simulink model "pll_wbsd_2"  (Simulink 7.4)
settings: Solver=ode45  StartTime=0.0  StopTime=1e-4  FixedStep=.01/(fr*N/M)  MaxStep=1/(50*fr*(N+f))  RelTol=1e-7  AbsTol=1e-4
PreLoadFcn:
  | fr=48e6,fi=2449e6,sen=200e6,N=51,f=0.125
undefined symbols (not defined in the file or in its folder): One, sen, sided
libraries: dspsigops x5, simulink_extras x2, dspswit3 x1, simulink x1, dspsnks4 x1, dsparch4 x1, commsynccomp2 x1
settings Model: Creator=Owner  LastModifiedBy=dbenson  SimulationMode=accelerator  BufferReuse=off
settings DataIOCC: LimitDataPoints=off  SaveOutput=off  SaveTime=off  SignalLoggingName=sigsOut
settings OptimizationCC: BlockReduction=off  BooleanDataType=off  InlineInvariantSignals=on  OptimizeBlockIOStorage=off  BufferReuse=off  ExpressionFolding=off  LocalBlockOutputs=off  InitFltsAndDblsToZero=on
settings DebuggingCC: SaveWithParameterizedLinksMsg=none  SignalResolutionControl=TryResolveAllWithWarning  SolverPrmCheckMsg=none  MultiTaskDSMMsg=warning  MultiTaskCondExecSysMsg=none  StrictBusMsg=None
settings HardwareCC: TargetUnknown=on
settings RTWCC: IncludeERTFirstTime=on
settings GRTTargetCC: TargetFcnLib=ansi_tfl_tmw.mat

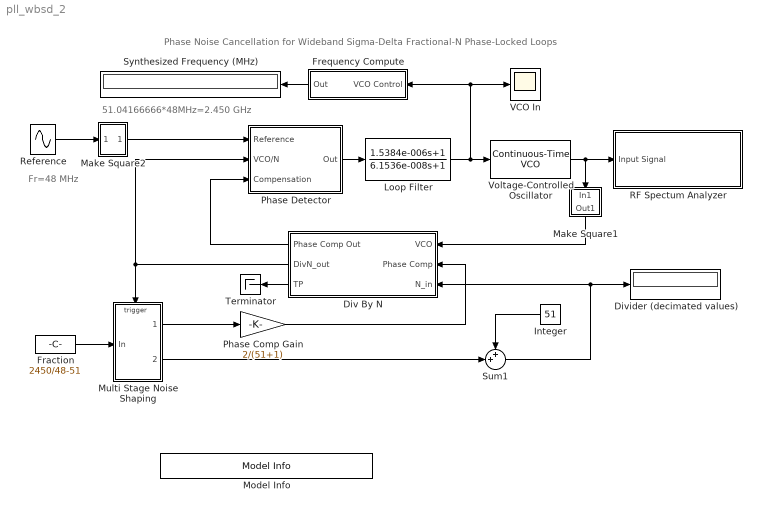
== system pll_wbsd_2 ==
  note: Phase Noise Cancellation for Wideband Sigma-Delta Fractional-N Phase-Locked Loops
  note: Fr=48 MHz
  note: 51.04166666*48MHz=2.450 GHz
  Div By N : Subsystem
  Divider (decimated values) : Display
      settings: Decimation=100
  Fraction : Constant  Value=2450/48-51  OutDataType=sfix(16)  OutScaling=2^0
  Frequency Compute : Subsystem
  Integer : Constant  Value=51  OutDataType=sfix(16)  OutScaling=2^0
  Loop Filter : TransferFcn  Numerator=[1.5384e-006 1]  Denominator=[6.1536e-008 1]
  Make Square1 : Subsystem
      mask Type: Make Square
      mask Description:
      | For input +ve values output is 1
      | For input -ve values output is 0
      mask Display: plot(0,0,100,100,[90,70,70,50,50,30,30,10,10],[20,20,40,40,20,20,40,40,20],[90,87,84,80,76,73,70,67,63,60,57,53,50,47,44,40,36,33,30,27,23,20,17,13,10],[70,65,63,62,63,65,70,75,77,78,77,75,70,65,63,62,63,65,70,75,77,78,77,75,70])
  Make Square2 : Subsystem
      mask Type: Make Square
      mask Description:
      | For input +ve values output is 1
      | For input -ve values output is 0
      mask Display: plot(0,0,100,100,[90,70,70,50,50,30,30,10,10],[20,20,40,40,20,20,40,40,20],[90,87,84,80,76,73,70,67,63,60,57,53,50,47,44,40,36,33,30,27,23,20,17,13,10],[70,65,63,62,63,65,70,75,77,78,77,75,70,65,63,62,63,65,70,75,77,78,77,75,70])
  Model Info : simulink/Model-Wide Utilities/Model Info  SystemSampleTime=-1  InitialBlockCM=none  BlockCM=none  Frame=on  DisplayStringWithTags=Copywrite 2005-2010 The MathWorks, Inc.  HorizontalTextAlignment=Center  LeftAlignmentValue=0.5  SourceBlockDiagram=pll_wbsd_2  TagMaxNumber=20
  Multi Stage Noise Shaping : Subsystem
  Phase Comp Gain : Gain  Gain=2/(51+1)  ParameterDataType=sfix(16)  ParameterScaling=2^0  OutDataType=sfix(16)  OutScaling=2^0  SaturateOnIntegerOverflow=on  OutDataTypeStr=Inherit: Same as input  ParamDataTypeStr=Inherit: Same as input
  Phase Detector : Subsystem
  RF Spectum Analyzer : Subsystem  Description=Spectrum Analyzer  mask{BW=10e6, Fc=2.450e9}
      mask prompts: BW "Bandwidth"; Fc "Center Freq"
      mask Display: fprintf('Spectrum Analyzer \n Fc=%7.2f MHz \n BW=%7.2f MHz',Fc/1e6,BW/1e6)
  Reference : Sin  Amplitude=1  Bias=0  Frequency=2*pi*(48e6)  Phase=0  Samples=10  SampleTime=0  Offset=0
  Sum1 : Sum  Inputs=++|  OutDataType=sfix(16)  OutScaling=2^0  SaturateOnIntegerOverflow=on  InputSameDT=on  OutDataTypeStr=Inherit: Same as first input
  Synthesized Frequency (MHz) : Display
      settings: Format=long_e  Decimation=401
  Terminator : Terminator
  VCO In : Scope
      settings: TickLabels=on  TimeRange=1e-005  YMin=0  YMax=0.015  MaxDataPoints=50000  Decimation=100
  Voltage-Controlled Oscillator : commsynccomp2/Continuous-Time VCO  SystemSampleTime=-1  Ac=1  Fc=fi  Kc=sen  Ph=0
  wires:
  Reference/1 -> Make Square2/1(In1)
  Frequency Compute/1(Out) -> Synthesized Frequency (MHz)/1
  Voltage-Controlled Oscillator/1 -> Make Square1/1(In1), RF Spectum Analyzer/1(Input Signal)
  Integer/1 -> Sum1/1
  Sum1/1 -> Div By N/3(N_in), Divider (decimated values)/1
  Multi Stage Noise Shaping/2(Sum 2) -> Sum1/2
  Div By N/1(Phase Comp Out) -> Phase Detector/3(Compensation)
  Multi Stage Noise Shaping/1(Sum 1) -> Phase Comp Gain/1
  Phase Comp Gain/1 -> Div By N/2(Phase Comp)
  Phase Detector/1(Out) -> Loop Filter/1
  Loop Filter/1 -> Voltage-Controlled Oscillator/1, VCO In/1, Frequency Compute/1(VCO Control)
  Make Square2/1(Out1) -> Phase Detector/1(Reference)
  Make Square1/1(Out1) -> Div By N/1(VCO)
  Div By N/2(DivN_out) -> Multi Stage Noise Shaping/Trigger, Phase Detector/2(VCO/N)
  Fraction/1 -> Multi Stage Noise Shaping/1(In)
  Div By N/3(TP) -> Terminator/1

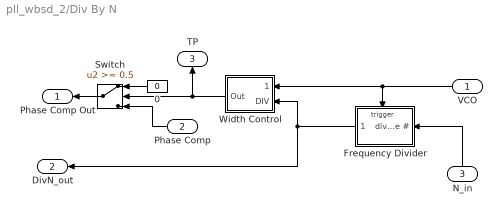
== system pll_wbsd_2/Div By N ==
  VCO : Inport  OutDataType=sfix(16)  OutScaling=2^0
  Phase Comp : Inport  Port=2  OutDataType=sfix(16)  OutScaling=2^0
  N_in : Inport  Port=3  OutDataType=sfix(16)  OutScaling=2^0
  0 : Constant  Value=0  OutDataType=sfix(16)  OutScaling=2^0
  Frequency Divider : Subsystem  TreatAsAtomicUnit=on
  Switch : Switch  Threshold=0.5  SaturateOnIntegerOverflow=on
  Width Control : Subsystem
  Phase Comp Out : Outport  OutDataType=sfix(16)  OutScaling=2^0
  DivN_out : Outport  Port=2  OutDataType=sfix(16)  OutScaling=2^0
  TP : Outport  Port=3  OutDataType=sfix(16)  OutScaling=2^0
  wires:
  Frequency Divider/1(" ") -> Width Control/2(DIV), DivN_out/1
  VCO/1 -> Width Control/1(VCO), Frequency Divider/Trigger
  0/1 -> Switch/1
  N_in/1 -> Frequency Divider/1("divide # ")
  Switch/1 -> Phase Comp Out/1
  Phase Comp/1 -> Switch/3
  Width Control/1(Out) -> Switch/2, TP/1

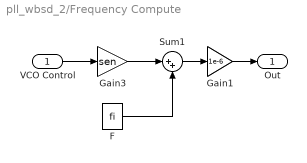
== system pll_wbsd_2/Frequency Compute ==
  VCO Control : Inport  OutDataType=sfix(16)  OutScaling=2^0
  F : Constant  Value=fi  OutDataType=sfix(16)  OutScaling=2^0
  Gain1 : Gain  Gain=1e-6  ParameterDataType=sfix(16)  ParameterScaling=2^0  OutDataType=sfix(16)  OutScaling=2^0  SaturateOnIntegerOverflow=on  OutDataTypeStr=Inherit: Same as input  ParamDataTypeStr=Inherit: Same as input
  Gain3 : Gain  Gain=sen  ParameterDataType=sfix(16)  ParameterScaling=2^0  OutDataType=sfix(16)  OutScaling=2^0  SaturateOnIntegerOverflow=on  OutDataTypeStr=Inherit: Same as input  ParamDataTypeStr=Inherit: Same as input
  Sum1 : Sum  Inputs=|++  OutDataType=sfix(16)  OutScaling=2^0  SaturateOnIntegerOverflow=on  InputSameDT=on  OutDataTypeStr=Inherit: Same as first input
  Out : Outport  OutDataType=sfix(16)  OutScaling=2^0
  wires:
  Sum1/1 -> Gain1/1
  F/1 -> Sum1/2
  Gain3/1 -> Sum1/1
  VCO Control/1 -> Gain3/1
  Gain1/1 -> Out/1

== system pll_wbsd_2/Make Square1 ==
  In1 : Inport  OutDataType=sfix(16)  OutScaling=2^0
  Constant : Constant  Value=0  OutDataType=sfix(16)  OutScaling=2^0
  Relational Operator : RelationalOperator  Operator=>  InputSameDT=on
  Out1 : Outport  OutDataType=sfix(16)  OutScaling=2^0
  wires:
  In1/1 -> Relational Operator/1
  Constant/1 -> Relational Operator/2
  Relational Operator/1 -> Out1/1

== system pll_wbsd_2/Make Square2 ==
  In1 : Inport  OutDataType=sfix(16)  OutScaling=2^0
  Constant : Constant  Value=0  OutDataType=sfix(16)  OutScaling=2^0
  Relational Operator : RelationalOperator  Operator=>  InputSameDT=on
  Out1 : Outport  OutDataType=sfix(16)  OutScaling=2^0
  wires:
  In1/1 -> Relational Operator/1
  Constant/1 -> Relational Operator/2
  Relational Operator/1 -> Out1/1

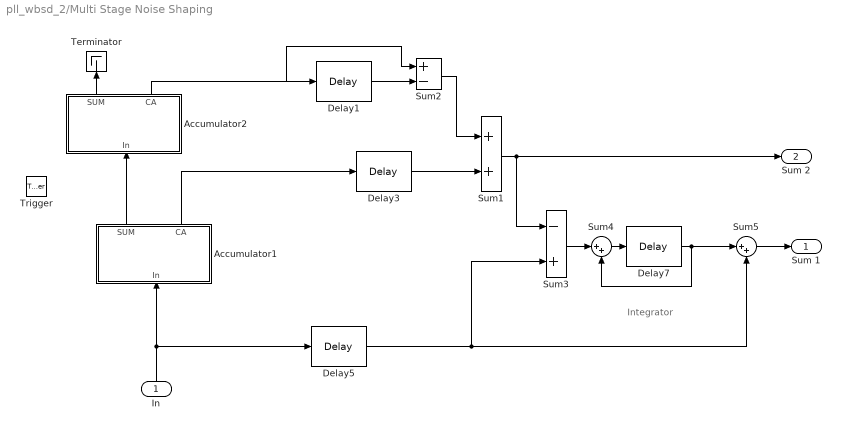
== system pll_wbsd_2/Multi Stage Noise Shaping ==
  note: Integrator
  In : Inport  OutDataType=sfix(16)  OutScaling=2^0
  Trigger : TriggerPort
  Accumulator1 : Subsystem  TreatAsAtomicUnit=on
  Accumulator2 : Subsystem  TreatAsAtomicUnit=on
  Delay{1,3,5,7} (4 alike) : dspsigops/Delay  dly_unit=Samples  delay=1  ic_detail=off  dif_ic_for_ch=off  dif_ic_for_dly=off  ic=0  reset_popup=None
  Sum1 : Sum  OutDataType=sfix(16)  OutScaling=2^0  SaturateOnIntegerOverflow=on  InputSameDT=on  OutDataTypeStr=Inherit: Same as first input
  Sum2 : Sum  Inputs=+-  OutDataType=sfix(16)  OutScaling=2^0  SaturateOnIntegerOverflow=on  InputSameDT=on  OutDataTypeStr=Inherit: Same as first input
  Sum3 : Sum  Inputs=-+  OutDataType=sfix(16)  OutScaling=2^0  SaturateOnIntegerOverflow=on  InputSameDT=on  OutDataTypeStr=Inherit: Same as first input
  Sum4 : Sum  Inputs=|++  OutDataType=sfix(16)  OutScaling=2^0  SaturateOnIntegerOverflow=on  InputSameDT=on  OutDataTypeStr=Inherit: Same as first input
  Sum5 : Sum  Inputs=|++  OutDataType=sfix(16)  OutScaling=2^0  SaturateOnIntegerOverflow=on  InputSameDT=on  OutDataTypeStr=Inherit: Same as first input
  Terminator : Terminator
  Sum 1 : Outport  OutDataType=sfix(16)  OutScaling=2^0
  Sum 2 : Outport  Port=2  OutDataType=sfix(16)  OutScaling=2^0
  wires:
  Delay7/1 -> Sum4/2, Sum5/1
  Delay5/1 -> Sum3/2, Sum5/2
  Sum4/1 -> Delay7/1
  Accumulator1/1(SUM) -> Accumulator2/1(In)
  Accumulator2/1(SUM) -> Terminator/1
  Sum3/1 -> Sum4/1
  Sum1/1 -> Sum3/1, Sum 2/1
  In/1 -> Accumulator1/1(In), Delay5/1
  Accumulator2/2(CA) -> Sum2/1, Delay1/1
  Delay3/1 -> Sum1/2
  Sum2/1 -> Sum1/1
  Accumulator1/2(CA) -> Delay3/1
  Delay1/1 -> Sum2/2
  Sum5/1 -> Sum 1/1

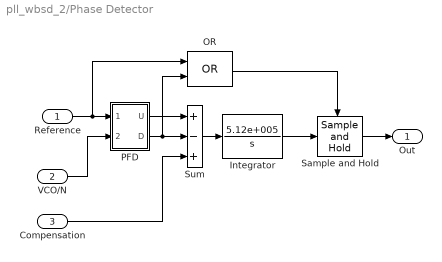
== system pll_wbsd_2/Phase Detector ==
  Reference : Inport  OutDataType=sfix(16)  OutScaling=2^0
  VCO/N : Inport  Port=2  OutDataType=sfix(16)  OutScaling=2^0
  Compensation : Inport  Port=3  OutDataType=sfix(16)  OutScaling=2^0
  Integrator : TransferFcn  Numerator=[5.12e+005]  Denominator=[1 0]
  OR : Logic  Operator=OR
  PFD : Subsystem
  Sample and Hold : dspsigops/Sample and Hold  SystemSampleTime=-1  trig=Rising edge  initCond=0  latchinput=off
  Sum : Sum  Inputs=+-+  OutDataType=sfix(16)  OutScaling=2^0  SaturateOnIntegerOverflow=on  InputSameDT=on  OutDataTypeStr=Inherit: Same as first input
  Out : Outport  OutDataType=sfix(16)  OutScaling=2^0
  wires:
  PFD/1(U) -> Sum/1
  OR/1 -> Sample and Hold/Trigger
  Reference/1 -> PFD/1(ref), OR/1
  PFD/2(D) -> Sum/2, OR/2
  Sum/1 -> Integrator/1
  Integrator/1 -> Sample and Hold/1
  VCO/N/1 -> PFD/2(var)
  Compensation/1 -> Sum/3
  Sample and Hold/1 -> Out/1

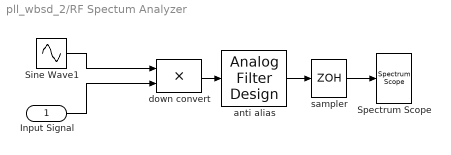
== system pll_wbsd_2/RF Spectum Analyzer ==
  Input Signal : Inport  OutDataType=sfix(16)  OutScaling=2^0
  Sine Wave1 : Sin  Amplitude=2*sqrt(2)  Bias=0  Frequency=2*pi*(Fc-BW/2)  Phase=-pi/2  Samples=10  SampleTime=0  Offset=0
  Spectrum Scope : dspsnks4/Spectrum Scope  DialogController=dspdialog.SpectrumScope  DialogControllerArgs=DataTag0  SystemSampleTime=-1  ScopeProperties=on  Domain=Frequency  HorizSpan=1  UseBuffer=on  BufferSize=256  Overlap=0  inpFftLenInherit=off  FFTlength=128  numAvg=1  DisplayProperties=off  AxisGrid=on  Memory=off  FrameNumber=on  AxisLegend=off  AxisZoom=off  OpenScopeAtSimStart=on  OpenScopeImmediately=off  FigPos=[4 30 389 221]  AxisProperties=off  XUnits=Hertz  XRange=One-sided ([0...Fs/2])  XDisplay=0  InheritXIncr=on  XIncr=1.0  XLabel=Samples  XLimit=Auto  YUnits=dBW  XMax=1  XMin=0  YLabel=dBW  LineProperties=off  wintypeSpecScope=Hann  RsSpecScope=50  betaSpecScope=5  winsampSpecScope=Periodic  XAxisParamsVer=6.9
      settings: YMin=-100  YMax=10
  anti alias : dsparch4/Analog Filter Design  method=Elliptic  filttype=Lowpass  N=8  Wlo=BW*2*pi  Whi=80  Rp=1  Rs=120
  down convert : Product  OutDataType=sfix(16)  OutScaling=2^0  SaturateOnIntegerOverflow=on  InputSameDT=on  OutDataTypeStr=Inherit: Same as first input
  sampler : ZeroOrderHold  SampleTime=1/(2.56*BW)
  wires:
  Sine Wave1/1 -> down convert/1
  sampler/1 -> Spectrum Scope/1
  anti alias/1 -> sampler/1
  down convert/1 -> anti alias/1
  Input Signal/1 -> down convert/2

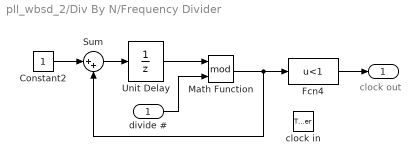
== system pll_wbsd_2/Div By N/Frequency Divider ==
  note: clock out
  "divide # " : Inport  OutDataType=sfix(16)  OutScaling=2^0  LatchByDelayingOutsideSignal=on
  clock in : TriggerPort
  Constant2 : Constant  OutDataType=sfix(16)  OutScaling=2^0
  Fcn4 : Fcn  Expr=u<1
  Math Function : Math  Operator=mod  OutDataType=sfix(16)  OutScaling=2^0  SaturateOnIntegerOverflow=on
  Sum : Sum  Inputs=|++  OutDataType=sfix(16)  OutScaling=2^0  SaturateOnIntegerOverflow=on  InputSameDT=on  OutDataTypeStr=Inherit: Same as first input
  Unit Delay : UnitDelay  SampleTime=-1
  " " : Outport  OutDataType=sfix(16)  OutScaling=2^0
  wires:
  "divide # "/1 -> Math Function/2
  Fcn4/1 -> " "/1
  Math Function/1 -> Fcn4/1, Sum/2
  Unit Delay/1 -> Math Function/1
  Constant2/1 -> Sum/1
  Sum/1 -> Unit Delay/1

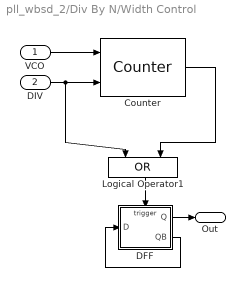
== system pll_wbsd_2/Div By N/Width Control ==
  VCO : Inport  OutDataType=sfix(16)  OutScaling=2^0
  DIV : Inport  Port=2  OutDataType=sfix(16)  OutScaling=2^0
  Counter : dspswit3/Counter  Direction=Up  CountEvent=Rising edge  CounterSize=User defined  MaxCount=255  InitialCount=0  Output=Hit  HitValue=27  ResetInput=on  SamplesPerFrame=1  Ts=1  CntDtype=double  HitDtype=Logical
  DFF : Subsystem
  Logical Operator1 : Logic  Operator=OR
  Out : Outport  OutDataType=sfix(16)  OutScaling=2^0
  wires:
  VCO/1 -> Counter/1
  DIV/1 -> Counter/2, Logical Operator1/1
  Counter/1 -> Logical Operator1/2
  DFF/1(Q) -> Out/1
  DFF/2(QB) -> DFF/1(D)
  Logical Operator1/1 -> DFF/Trigger

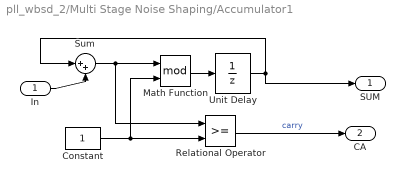
== system pll_wbsd_2/Multi Stage Noise Shaping/Accumulator1 ==
  In : Inport  OutDataType=sfix(16)  OutScaling=2^0
  Constant : Constant  OutDataType=sfix(16)  OutScaling=2^0
  Math Function : Math  Operator=mod  OutDataType=sfix(16)  OutScaling=2^0  SaturateOnIntegerOverflow=on
  Relational Operator : RelationalOperator  InputSameDT=on
  Sum : Sum  Inputs=|++  OutDataType=sfix(16)  OutScaling=2^0  SaturateOnIntegerOverflow=on  InputSameDT=on  OutDataTypeStr=Inherit: Same as first input
  Unit Delay : UnitDelay  SampleTime=-1
  SUM : Outport  OutDataType=sfix(16)  OutScaling=2^0
  CA : Outport  Port=2  OutDataType=sfix(16)  OutScaling=2^0
  wires:
  In/1 -> Sum/2
  Relational Operator/1 -> CA/1  "carry"
  Unit Delay/1 -> SUM/1, Sum/1
  Constant/1 -> Relational Operator/2, Math Function/2
  Math Function/1 -> Unit Delay/1
  Sum/1 -> Math Function/1, Relational Operator/1

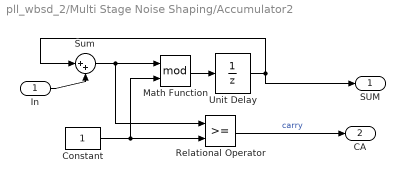
== system pll_wbsd_2/Multi Stage Noise Shaping/Accumulator2 ==
  In : Inport  OutDataType=sfix(16)  OutScaling=2^0
  Constant : Constant  OutDataType=sfix(16)  OutScaling=2^0
  Math Function : Math  Operator=mod  OutDataType=sfix(16)  OutScaling=2^0  SaturateOnIntegerOverflow=on
  Relational Operator : RelationalOperator  InputSameDT=on
  Sum : Sum  Inputs=|++  OutDataType=sfix(16)  OutScaling=2^0  SaturateOnIntegerOverflow=on  InputSameDT=on  OutDataTypeStr=Inherit: Same as first input
  Unit Delay : UnitDelay  SampleTime=-1
  SUM : Outport  OutDataType=sfix(16)  OutScaling=2^0
  CA : Outport  Port=2  OutDataType=sfix(16)  OutScaling=2^0
  wires:
  Sum/1 -> Relational Operator/1, Math Function/1
  Math Function/1 -> Unit Delay/1
  Constant/1 -> Math Function/2, Relational Operator/2
  Unit Delay/1 -> Sum/1, SUM/1
  Relational Operator/1 -> CA/1  "carry"
  In/1 -> Sum/2

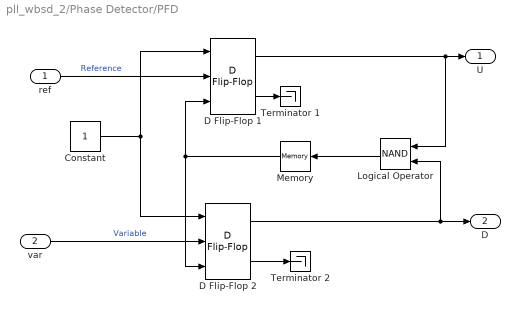
== system pll_wbsd_2/Phase Detector/PFD ==
  ref : Inport  OutDataType=sfix(16)  OutScaling=2^0
  var : Inport  Port=2  OutDataType=sfix(16)  OutScaling=2^0
  Constant : Constant  OutDataType=sfix(16)  OutScaling=2^0
  D Flip-Flop 1 : simulink_extras/Flip Flops/D Flip-Flop  SystemSampleTime=-1
  D Flip-Flop 2 : simulink_extras/Flip Flops/D Flip-Flop  SystemSampleTime=-1
  Logical Operator : Logic  Operator=NAND
  Memory : Memory
  Terminator 1 : Terminator
  Terminator 2 : Terminator
  U : Outport  OutDataType=sfix(16)  OutScaling=2^0
  D : Outport  Port=2  OutDataType=sfix(16)  OutScaling=2^0
  wires:
  var/1 -> D Flip-Flop 2/2  "Variable"
  D Flip-Flop 1/2 -> Terminator 1/1
  D Flip-Flop 2/2 -> Terminator 2/1
  ref/1 -> D Flip-Flop 1/2  "Reference"
  Constant/1 -> D Flip-Flop 1/1, D Flip-Flop 2/1
  Memory/1 -> D Flip-Flop 1/3, D Flip-Flop 2/3
  D Flip-Flop 1/1 -> U/1, Logical Operator/1
  D Flip-Flop 2/1 -> D/1, Logical Operator/2
  Logical Operator/1 -> Memory/1

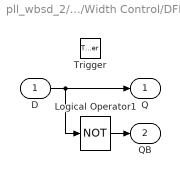
== system pll_wbsd_2/Div By N/Width Control/DFF ==
  D : Inport  OutDataType=sfix(16)  OutScaling=2^0  LatchByDelayingOutsideSignal=on
  Trigger : TriggerPort
  Logical Operator1 : Logic  Operator=NOT
  Q : Outport  OutDataType=sfix(16)  OutScaling=2^0
  QB : Outport  Port=2  OutDataType=sfix(16)  OutScaling=2^0
  wires:
  D/1 -> Q/1, Logical Operator1/1
  Logical Operator1/1 -> QB/1
